simulink model "reichardt_array_EMD_fly"  (R2018b)
settings: Solver=ode45  StartTime=0.0  StopTime=setStopTime  FixedStep=0.0005  RelTol=1e-3  EnableMultiTasking=on
model workspace (MAT data in the model file):
  bodyAmp = 0
  bodyPhase = 0
  freq = 75.3982236862
  headAmp = 1.28658400111
  headPhase = -0.267444430956
  imageData = [0.00228480667088 0.00685422825671 0.0114230745906 0.0159909622235 0.0205575077854 0.0251223280162 0.0296850397975 0.0342452601838 0.0388026064343 0.0433566960441 0.0479071467754 0.0524535766893 ... (8204 elements, 1x8204)]
  outputTimeList = [1 1.00083333333 1.00166666667 1.0025 1.00333333333 1.00416666667 1.005 1.00583333333 1.00666666667 1.0075 1.00833333333 1.00916666667 ... (101 elements, 1x101)]
  setStopTime = 1.08333333333
  stimAmp = 15
  temporalFilt = 0.035
  timeConstant = 0.035
undefined symbols (not defined in the file or in its folder): lp_a, lp_b
libraries: visionsources x1
(part 2 of 2)

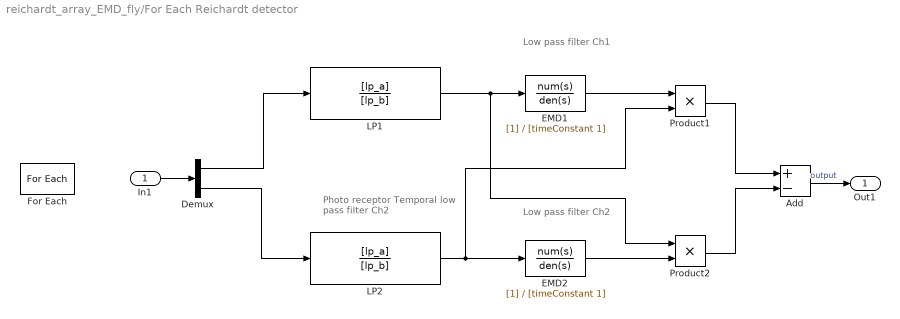
== system reichardt_array_EMD_fly/For Each Reichardt detector ==
  note: Photo receptor
      | Temporal low pass filter
      | Ch2
  note: Low pass filter
      | Ch1
  note: Low pass filter
      | Ch2
  In1 : Inport  Partition=on  PartitionDimension=1  PartitionWidth=1  PartitionOffset=0
  Add : Sum  Inputs=+-
  Demux : Demux  Outputs=2
  EMD1 : TransferFcn  Denominator=[timeConstant 1]
  EMD2 : TransferFcn  Denominator=[timeConstant 1]
  For Each : ForEach  DisableCoverage=on  IndexMode=One-based
  LP1 : TransferFcn  Numerator=[lp_a]  Denominator=[lp_b]
  LP2 : TransferFcn  Numerator=[lp_a]  Denominator=[lp_b]
  Product1 : Product  RndMeth=Zero
  Product2 : Product  RndMeth=Zero
  Out1 : Outport  ConcatenationDimension=1
  wires:
  EMD1/1 -> Product1/1
  Product1/1 -> Add/1
  Product2/1 -> Add/2
  EMD2/1 -> Product2/2
  Add/1 -> Out1/1  "output"
  In1/1 -> Demux/1
  LP2/1 -> Product1/2, EMD2/1
  LP1/1 -> EMD1/1, Product2/1
  Demux/1 -> LP1/1
  Demux/2 -> LP2/1

== matlab function reichardt_array_EMD_fly/sampleImage ==
  data: imageData input; intensity output double size=360,2; seenAngle input
function intensity = fcn(imageData,seenAngle)
%#codegen

imageWidth = length(imageData);

% Subsample with resolution of compound eye
sampleCoord = 0:359;
sampleCoord = sampleCoord + seenAngle;
sampleCoord = mod(sampleCoord,360);
temp        = interp1(linspace(0,360,imageWidth),imageData,sampleCoord);

% Create output signals
intensity = [temp(:), circshift(temp(:),-1)];
